simulink model "QuadcopterEMSubs"  (R2023b)
settings: Solver=VariableStepAuto  StartTime=0.0  StopTime=10.0  RelTol=1e-3
libraries: fl_lib x15, nesl_utility x11, sdl_lib x4, ee_lib x4, batteryecm_lib x1
(part 2 of 2)

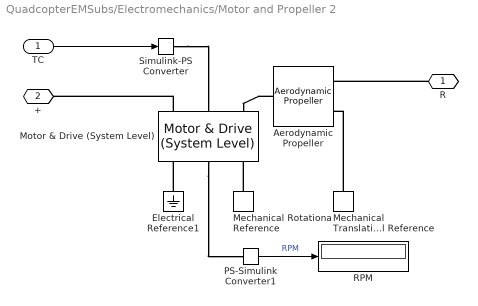
== system QuadcopterEMSubs/Electromechanics/Motor and Propeller 2 ==
  TC : Inport
  Aerodynamic Propeller : sdl_lib/Engines & Motors/Aerodynamic Propeller  parameterization=sdl.enum.PropellerParameterization.Constant  pitch_type=foundation.enum.constant_controlled.constant  direction=sdl.enum.PropellerDirection.Negative  root_pitch=0 deg  D=D m  kt_const=kT  kp_const=kP  kt_poly_fixed=[.002, .0006, -.0509, .0617]  kp_poly_fixed=[-.0752, .0577, -.0622, .16]  pitch_angle_TLU=[-15, 15, 25, 35, 45] deg  kt_poly_TLU=[.0002, -.00041, -.036, .03; .00026, -.00056, -.048, .04; .002, .00063, -.051, .062; .0014, -.0016, -.048, .087; .00087, -.0036, -.041, .12]  kp_poly_TLU=[-.1, .031, .0055, .088; -.081, -.025, .0044, .07; -.075, .058, -.062, .16; -.052, .065, -.08, .3; -.031, .057, -.069, .4]  J_TLU=[.01, .3, .625, 1.55, 2, 2.6]  kt_TLU_1D=[.0614, .0473, .0318, -.0127, -.0343, -.063]  kp_TLU_1D=[.1496, .1314, .116, -.0521, -.1503, -.2813]  kt_TLU_2D=[.00019, .013, .0048, -.017, -.03, -.045; .00039, .025, .0096, -.037, -.06, -.09; .00061, .047, .032, -.013, -.034, -.063; .00086, .072, .057, .014, -.0076, -.036; .12, .104, .09, .049, .029, .0019]  kp_TLU_2D=[.029, .029, .016, .06, .009, -.16; .059, .054, .031, -.12, -.19, -.29; .15, .13, .12, -.052, -.15, -.28; .26, .24, .22, .097, -.04, -.25; .39, .39, .38, .32, .24, .062]  beta_TLU=linspace(0, 360, 10) deg  Ct_TLU_1D=0.035 * sind(linspace(0, 360, 10) - 200)  Cq_TLU_1D=0.010 * sind(linspace(0, 360, 10) - 200)  Ct_TLU_2D=[0.01 * sind(linspace(0, 360, 10) - 200); 0.020 * sind(linspace(0, 360, 10) - 200); 0.035 * sind(linspace(0, 360, 10) - 200); 0.04 * sind(linspace(0, 360, 10) - 200); 0.06 * sind(linspace(0, 360, 10) - 200)]  Cq_TLU_2D=[0.0005 * sind(linspace(0, 360, 10) - 200); 0.0015 * sind(linspace(0, 360, 10) - 200); 0.0025 * sind(linspace(0, 360, 10) - 200); 0.0035 * sind(linspace(0, 360, 10) - 200); 0.0045 * sind(linspace(0, 360, 10) - 200)]  n_blades=2  n_blade_discretization=20  radial_TLU=[.05, .09, .13, .19, .25, .32, .39, .45, .52, .58, .65, .72, 1]  twist_TLU=[48.55, 48.55, 48.55, 48.55, 38.9, 32.39, 27.05, 21.76, 16.74, 12.41, 8.57, 5.52, .034] deg  chord_TLU=[.029, .031, .034, .037, .038, .036, .034, .033, .03, .028, .026, .024, .012]  alpha_TLU=[-180, -169, -161, -143, -39, -28 : -23, -16 : -13, -3, 7 : 17, 21, 35, 36, 60, 120, 144, 160, 169, 180] deg  Cl_TLU=[0, 0, 0, .0038, .0038, .0038, .0044, .0059, .0059, .0063, .0063, .006, .006; 0, 0, 0, .4279, .4367, .4367, .5701, .7465, .7465, .794, .794, .7565, .7565; 0, 0, 0, .6251, .6405, .6405, .6716, .6871, .6871, .6646, .6646, .653, .653; 0, 0, 0, .77, .7939, .7939, .8365, .8507, .8507, .8182, .8182, .8031, .8031; 0, 0, 0, -.8855, -.8888, -.8888, -.8956, -.8987, -.8987, -.8756, -.8756, -.8664, -.8664; 0, 0, 0, -.8164, -.8237, -.8237, -.8446, -.8396, -.8396, -.8173, -.8173, -.8311, -.8311; 0, 0, 0, -.8035, -.8107, -.8107, -.8387, -.8268, -.8268, -.8062, -.8062, -.837, -.837; 0, 0, 0, -.7899, -.7969, -.7969, -.8342, -.8141, -.8141, -.7967, -.7967, -.8448, -.8448; 0, 0, 0, -.7759, -.7829, -.7829, -.8321, -.8021, -.8021, -.7907, -.7907, -.8538, -.8538; 0, 0, 0, -.7597, -.7667, -.7667, -.854, -.7916, -.7916, -.7946, -.7946, -.8715, -.8715; 0, 0, 0, -.7426, -.7496, -.7496, -.8847, -.7891, -.7891, -.8061, -.8061, -.8916, -.8916; 0, 0, 0, -.5682, -.5992, -.5992, -1.2502, -.9071, -.9071, -1.0018, -1.0018, -1.1131, -1.1131; 0, 0, 0, -.5309, -.5773, -.5773, -1.2818, -.9342, -.9342, -1.036, -1.036, -1.1036, -1.1036; 0, 0, 0, -.4907, -.5574, -.5574, -1.2049, -.9612, -.9612, -1.0439, -1.0439, -1.075, -1.075; 0, 0, 0, -.4485, -.5374, -.5374, -1.1187, -.9852, -.9852, -1.0006, -1.0006, -1.0074, -1.0074; 0, 0, 0, .0053, -.2277, -.2277, -.1089, .0596, .0596, .1552, .1552, .0974, .0974; 0, 0, 0, 1.093, 1.1442, 1.1442, 1.2067, 1.2616, 1.2616, 1.2898, 1.2898, 1.1872, 1.1872; 0, 0, 0, 1.2011, 1.2696, 1.2696, 1.3122, 1.3414, 1.3414, 1.3628, 1.3628, 1.2629, 1.2629; 0, 0, 0, 1.2944, 1.3764, 1.3764, 1.3958, 1.4048, 1.4048, 1.4045, 1.4045, 1.331, 1.331; 0, 0, 0, 1.3733, 1.483, 1.483, 1.4631, 1.4421, 1.4421, 1.3507, 1.3507, 1.3853, 1.3853; 0, 0, 0, 1.4289, 1.5767, 1.5767, 1.5156, 1.3648, 1.3648, 1.2843, 1.2843, 1.4168, 1.4168; 0, 0, 0, 1.4765, 1.6474, 1.6474, 1.5515, 1.2718, 1.2718, 1.2722, 1.2722, 1.4354, 1.4354; 0, 0, 0, 1.5166, 1.7035, 1.7035, 1.4574, 1.246, 1.246, 1.273, 1.273, 1.4517, 1.4517; 0, 0, 0, 1.5662, 1.7108, 1.7108, 1.3502, 1.2569, 1.2569, 1.272, 1.272, 1.4472, 1.4472; 0, 0, 0, 1.6172, 1.6861, 1.6861, 1.3319, 1.2727, 1.2727, 1.2756, 1.2756, 1.4453, 1.4453; 0, 0, 0, 1.6518, 1.6448, 1.6448, 1.3288, 1.2899, 1.2899, 1.2853, 1.2853, 1.4478, 1.4478; 0, 0, 0, 1.6837, 1.5939, 1.5939, 1.3215, 1.305, 1.305, 1.3065, 1.3065, 1.4376, 1.4376; 0, 0, 0, 1.8117, 1.5649, 1.5649, 1.4361, 1.359, 1.359, 1.3219, 1.3219, 1.3984, 1.3984; 0, 0, 0, 1.9292, 1.5442, 1.5442, 1.2641, 1.0661, 1.0661, .9471, .9471, .8, .8; 0, 0, 0, 1.9291, 1.5451, 1.5451, 1.2647, 1.0667, 1.0667, .9484, .9484, .8003, .8003; 0, 0, 0, 1.3197, 1.0944, 1.0944, .93, .8084, .8084, .7386, .7386, .6549, .6549; 0, 0, 0, -.5504, -.5764, -.5764, -.5794, -.5974, -.5974, -.6384, -.6384, -.6414, -.6414; 0, 0, 0, -.7967, -.8179, -.8179, -.815, -.8265, -.8265, -.8695, -.8695, -.8727, -.8727; 0, 0, 0, -.6625, -.6755, -.6755, -.6718, -.678, -.678, -.71, -.71, -.7129, -.7129; 0, 0, 0, -.4372, -.4449, -.4449, -.5659, -.7443, -.7443, -.797, -.797, -.7602, -.7602; 0, 0, 0, -.0005, -.0005, -.0005, -.0005, -.0007, -.0007, -.0008, -.0008, -.0007, -.0007]  Cd_TLU=[.5, .5, .35, .0113, .0094, .0094, .0087, .0065, .0065, .0057, .0057, .0052, .0052; .5, .5, .35, .1226, .1192, .1192, .111, .1087, .1087, .1087, .1087, .1096, .1096; .5, .5, .35, .2813, .2754, .2754, .265, .2622, .2622, .2588, .2588, .2588, .2588; .5, .5, .35, .6981, .6956, .6956, .6919, .6916, .6916, .6764, .6764, .6716, .6716; .5, .5, .35, .6005, .6252, .6252, .6685, .6821, .6821, .654, .654, .6398, .6398; .5, .5, .35, .351, .3709, .3709, .4054, .4161, .4161, .3965, .3965, .3833, .3833; .5, .5, .35, .3293, .3486, .3486, .3824, .3927, .3927, .3737, .3737, .3588, .3588; .5, .5, .35, .3079, .3266, .3266, .3597, .3693, .3693, .3508, .3508, .3341, .3341; .5, .5, .35, .2866, .3047, .3047, .3375, .346, .346, .3275, .3275, .3091, .3091; .5, .5, .35, .2658, .2834, .2834, .3163, .3228, .3228, .3033, .3033, .2835, .2835; .5, .5, .35, .2456, .2625, .2625, .2962, .2991, .2991, .2782, .2782, .2577, .2577; .5, .5, .35, .129, .1313, .1313, .1766, .1275, .1275, .096, .096, .0806, .0806; .5, .5, .35, .119, .1157, .1157, .1621, .1039, .1039, .0709, .0709, .0555, .0555; .5, .5, .35, .1107, .1011, .1011, .143, .0807, .0807, .0494, .0494, .0303, .0303; .5, .5, .35, .1041, .0877, .0877, .123, .0586, .0586, .034, .034, .0152, .0152; .5, .5, .35, .0307, .0145, .0145, .0089, .0068, .0068, .0058, .0058, .0065, .0065; .5, .5, .35, .0156, .0115, .0115, .0106, .013, .013, .013, .013, .0112, .0112; .5, .5, .35, .0194, .0119, .0119, .0123, .0151, .0151, .0146, .0146, .0123, .0123; .5, .5, .35, .0268, .0132, .0132, .0153, .0178, .0178, .0177, .0177, .0135, .0135; .5, .5, .35, .0381, .0154, .0154, .0188, .0252, .0252, .0248, .0248, .0148, .0148; .5, .5, .35, .0563, .019, .019, .0248, .0406, .0406, .0339, .0339, .0365, .0365; .5, .5, .35, .0794, .0262, .0262, .0359, .0587, .0587, .0457, .0457, .0595, .0595; .5, .5, .35, .1104, .0384, .0384, .0602, .077, .077, .0619, .0619, .0823, .0823; .5, .5, .35, .1435, .0591, .0591, .0907, .0982, .0982, .0792, .0792, .1047, .1047; .5, .5, .35, .1813, .0944, .0944, .1213, .1201, .1201, .0973, .0973, .1269, .1269; .5, .5, .35, .2217, .1343, .1343, .1565, .1416, .1416, .1154, .1154, .1491, .1491; .5, .5, .35, .2649, .1779, .1779, .1878, .1632, .1632, .1352, .1352, .1711, .1711; .5, .5, .35, .4382, .3418, .3418, .2921, .2513, .2513, .2194, .2194, .2573, .2573; .5, .5, .35, 1.0687, .884, .884, .7413, .6526, .6526, .6107, .6107, .5307, .5307; .5, .5, .35, 1.1128, .9207, .9207, .7724, .6799, .6799, .6362, .6362, .5527, .5527; .5, .5, .35, 1.8354, 1.5718, 1.5718, 1.3636, 1.232, 1.232, 1.1782, 1.1782, 1.0678, 1.0678; .5, .5, .35, 1.1876, 1.1903, 1.1903, 1.1775, 1.1722, 1.1722, 1.207, 1.207, 1.2112, 1.2112; .5, .5, .35, .7009, .6946, .6946, .6841, .6742, .6742, .6875, .6875, .6898, .6898; .5, .5, .35, .3164, .3083, .3083, .3017, .2929, .2929, .2939, .2939, .2948, .2948; .5, .5, .35, .1294, .1254, .1254, .1229, .1168, .1168, .1143, .1143, .1146, .1146; .5, .5, .35, .0601, .0405, .0405, .0265, .0201, .0201, .0184, .0184, .0197, .0197]  interp_method=simscape.enum.interpolation.linear  extrap_method=simscape.enum.extrapolation.linear  density_spec=foundation.enum.constant_variable.constant  rho=1.225 kg/m^3  rotational_ports=sdl.enum.ConnectionType.Conserving  translational_ports=sdl.enum.ConnectionType.Conserving  model_inertia=true  propeller_inertia=J kg*m^2  propeller_mass=m g  efficiency_sensor=false  n_thr=0.001 Hz  k_thr=0.001  P_thr=0.01 W  operation_check=simscape.enum.assert.action.warn  expose_port_C=0  w_specify=off  w_priority=None  w=0 rad/s  w_nominal_specify=off  w_nominal_unit=rad/s  w_nominal_value=1  Q_specify=off  Q_priority=None  Q=0 N*m  Q_nominal_specify=off  Q_nominal_unit=N*m  Q_nominal_value=1  v_specify=off  v_priority=None  v=0 m/s  v_nominal_specify=off  v_nominal_unit=m/s  v_nominal_value=1  thrust_specify=off  thrust_priority=None  thrust=0 N  thrust_nominal_specify=off  thrust_nominal_unit=N  thrust_nominal_value=1
      settings: InternalSimscapePortConfiguration="{\"Bottom\":[],\"Left\":[{\"id\":\"R1\",\"label\":\"R1\",\"type\":\"foundation.mechanical.rotational.rotational\"}],\"Right\":[{\"id\":\"R2\",\"label\":\"R2\",\"type\":\"foundation.mechanical.translational.translational\"},{\"id\":\"C2\",\"label\":\"C2\",\"type\":\"foundation.mechanical.translational.translational\"}],\"Top\":[]}"
  Electrical Reference1 : fl_lib/Electrical/Electrical Elements/Electrical Reference
  Mechanical Rotational Reference : fl_lib/Mechanical/Rotational Elements/Mechanical Rotational Reference
  Mechanical Translational Reference : fl_lib/Mechanical/Translational Elements/Mechanical Translational Reference
  Motor & Drive (System Level) : ee_lib/Electromechanical/Motor & Drive (System Level)  torque_speed_param=ee.enum.electromech.envelope.torque_power  overtorque_param=ee.enum.electromech.overtorque.no  T_t=[.09, .08, .07, 0] N*m  T_t_intermittent=[.36, .32, .28, 0] N*m  T_t_2D=[.09, .09, .09; .08, .08, .08; .07, .07, .07; 0, 0, 0] N*m  T_t_intermittent_2D=[.36, .36, .36; .32, .32, .32; .28, .28, .28; 0, 0, 0] N*m  w_t=[0, 3750, 7500, 8000] rpm  vdc_t=[6, 12, 24] V  torque_max=1 mN*m  power_max=3 W  torque_max_intermittent=0.4 N*m  power_max_intermittent=120 W  time_overtorque=30 s  time_recover=60 s  Tc=0.02 s  EnableSwitch=simscape.enum.onoff.off  losses_param=1  eff=74  w_eff=3e4 rpm  T_eff=1 mN*m  Piron=0 W  Pbase=0 W  w_eff_vec=[-8000, -4000, 0, 4000, 8000] rpm  T_eff_vec=[0, .03, .06, .09] N*m  v_eff_vec=[100, 250, 400] V  losses_mat=[1.49, 1.67, 2.21, 3.1; .42, .69, 1.14, 2.03; .06, .24, .78, 1.68; .42, .69, 1.14, 2.03; 1.49, 1.67, 2.21, 3.1] W  efficiency_mat=[95, 95, 95, 95; 95, 95, 95, 95; 95, 95, 95, 95; 95, 95, 95, 95; 95, 95, 95, 95]  losses_mat_3D=ones(5, 4, 3) W  efficiency_mat_3D=95 * ones(5, 4, 3)  Res=0 Ohm  enable_fault=simscape.enum.onoff.off  fault_condition=1  fault_threshold=0.5  J=8e-9 kg*m^2  lam=2.5e-8 N*m*s/rad  speed0=0 rpm  faulted_specify=off  faulted_priority=None  faulted=0  faulted_nominal_specify=off  faulted_nominal_unit=1  faulted_nominal_value=1  isSwitchedOff_specify=off  isSwitchedOff_priority=None  isSwitchedOff=0  isSwitchedOff_nominal_specify=off  isSwitchedOff_nominal_unit=1  isSwitchedOff_nominal_value=1  torqueLimitContinuous_specify=off  torqueLimitContinuous_priority=None  torqueLimitContinuous=0 N*m  torqueLimitContinuous_nominal_specify=off  torqueLimitContinuous_nominal_unit=N*m  torqueLimitContinuous_nominal_value=1  alpha=3.93e-3 1/K  Tmeas=25 degC  Tmeas2=125 degC  losses_mat_T2=[1.49, 1.74, 2.49, 3.74; .42, .67, 1.42, 2.67; .06, .31, 1.06, 2.31; .42, .67, 1.42, 2.67; 1.49, 1.74, 2.49, 3.74] W  efficiency_mat_T2=[95, 95, 95, 95; 95, 95, 95, 95; 95, 95, 95, 95; 95, 95, 95, 95; 95, 95, 95, 95]  losses_mat_3D_T2=ones(5, 4, 3) W  efficiency_mat_3D_T2=95 * ones(5, 4, 3)  thermal_mass=100 J/K  initial_temperature=25 degC
  PS-Simulink Converter1 : nesl_utility/PS-Simulink Converter  PhysicalDomain=network_engine_domain  SubClassName=ps_output  LeftPortType=input  RightPortType=output  PseudoPeriodic=off  Frequencies=[]  VectorFormat=inherit  Unit=rpm  AffineConversion=off
  RPM : Display
  Simulink-PS Converter : nesl_utility/Simulink-PS Converter  PhysicalDomain=network_engine_domain  SubClassName=ps_input  LeftPortType=input  RightPortType=output  PseudoPeriodic=off  Frequencies=[]  NoiseDistribution=none  NoiseParameters=[]  Unit=mN*m  AffineConversion=off  FilteringAndDerivatives=provide  SimscapeFilterOrder=1  InputFilterTimeConstant=0.001  UdotUserProvided=0
  R : PMIOPort  Side=Right
  + : PMIOPort  Port=2  Side=Left
  wires:
  TC/1 -> Simulink-PS Converter/1
  PS-Simulink Converter1/1 -> RPM/1  "RPM"
  connections:
  Mechanical Rotational Reference/LConn1 -- Motor & Drive (System Level)/RConn3
  Electrical Reference1/LConn1 -- Motor & Drive (System Level)/RConn1
  Aerodynamic Propeller/LConn1 -- Motor & Drive (System Level)/LConn3
  Motor & Drive (System Level)/RConn2 -- PS-Simulink Converter1/LConn1
  Mechanical Translational Reference/LConn1 -- Aerodynamic Propeller/RConn2
  R/RConn1 -- Aerodynamic Propeller/RConn1
  Simulink-PS Converter/RConn1 -- Motor & Drive (System Level)/LConn2
  Motor & Drive (System Level)/LConn1 -- +/RConn1

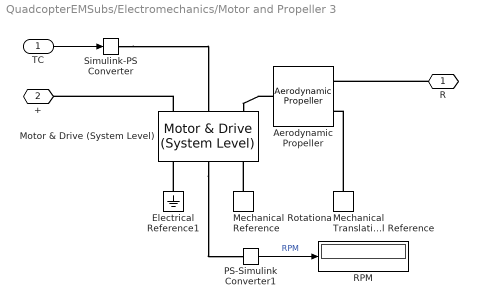
== system QuadcopterEMSubs/Electromechanics/Motor and Propeller 3 ==
  TC : Inport
  Aerodynamic Propeller : sdl_lib/Engines & Motors/Aerodynamic Propeller  parameterization=sdl.enum.PropellerParameterization.Constant  pitch_type=foundation.enum.constant_controlled.constant  direction=sdl.enum.PropellerDirection.Positive  root_pitch=0 deg  D=D m  kt_const=kT  kp_const=kP  kt_poly_fixed=[.002, .0006, -.0509, .0617]  kp_poly_fixed=[-.0752, .0577, -.0622, .16]  pitch_angle_TLU=[-15, 15, 25, 35, 45] deg  kt_poly_TLU=[.0002, -.00041, -.036, .03; .00026, -.00056, -.048, .04; .002, .00063, -.051, .062; .0014, -.0016, -.048, .087; .00087, -.0036, -.041, .12]  kp_poly_TLU=[-.1, .031, .0055, .088; -.081, -.025, .0044, .07; -.075, .058, -.062, .16; -.052, .065, -.08, .3; -.031, .057, -.069, .4]  J_TLU=[.01, .3, .625, 1.55, 2, 2.6]  kt_TLU_1D=[.0614, .0473, .0318, -.0127, -.0343, -.063]  kp_TLU_1D=[.1496, .1314, .116, -.0521, -.1503, -.2813]  kt_TLU_2D=[.00019, .013, .0048, -.017, -.03, -.045; .00039, .025, .0096, -.037, -.06, -.09; .00061, .047, .032, -.013, -.034, -.063; .00086, .072, .057, .014, -.0076, -.036; .12, .104, .09, .049, .029, .0019]  kp_TLU_2D=[.029, .029, .016, .06, .009, -.16; .059, .054, .031, -.12, -.19, -.29; .15, .13, .12, -.052, -.15, -.28; .26, .24, .22, .097, -.04, -.25; .39, .39, .38, .32, .24, .062]  beta_TLU=linspace(0, 360, 10) deg  Ct_TLU_1D=0.035 * sind(linspace(0, 360, 10) - 200)  Cq_TLU_1D=0.010 * sind(linspace(0, 360, 10) - 200)  Ct_TLU_2D=[0.01 * sind(linspace(0, 360, 10) - 200); 0.020 * sind(linspace(0, 360, 10) - 200); 0.035 * sind(linspace(0, 360, 10) - 200); 0.04 * sind(linspace(0, 360, 10) - 200); 0.06 * sind(linspace(0, 360, 10) - 200)]  Cq_TLU_2D=[0.0005 * sind(linspace(0, 360, 10) - 200); 0.0015 * sind(linspace(0, 360, 10) - 200); 0.0025 * sind(linspace(0, 360, 10) - 200); 0.0035 * sind(linspace(0, 360, 10) - 200); 0.0045 * sind(linspace(0, 360, 10) - 200)]  n_blades=2  n_blade_discretization=20  radial_TLU=[.05, .09, .13, .19, .25, .32, .39, .45, .52, .58, .65, .72, 1]  twist_TLU=[48.55, 48.55, 48.55, 48.55, 38.9, 32.39, 27.05, 21.76, 16.74, 12.41, 8.57, 5.52, .034] deg  chord_TLU=[.029, .031, .034, .037, .038, .036, .034, .033, .03, .028, .026, .024, .012]  alpha_TLU=[-180, -169, -161, -143, -39, -28 : -23, -16 : -13, -3, 7 : 17, 21, 35, 36, 60, 120, 144, 160, 169, 180] deg  Cl_TLU=[0, 0, 0, .0038, .0038, .0038, .0044, .0059, .0059, .0063, .0063, .006, .006; 0, 0, 0, .4279, .4367, .4367, .5701, .7465, .7465, .794, .794, .7565, .7565; 0, 0, 0, .6251, .6405, .6405, .6716, .6871, .6871, .6646, .6646, .653, .653; 0, 0, 0, .77, .7939, .7939, .8365, .8507, .8507, .8182, .8182, .8031, .8031; 0, 0, 0, -.8855, -.8888, -.8888, -.8956, -.8987, -.8987, -.8756, -.8756, -.8664, -.8664; 0, 0, 0, -.8164, -.8237, -.8237, -.8446, -.8396, -.8396, -.8173, -.8173, -.8311, -.8311; 0, 0, 0, -.8035, -.8107, -.8107, -.8387, -.8268, -.8268, -.8062, -.8062, -.837, -.837; 0, 0, 0, -.7899, -.7969, -.7969, -.8342, -.8141, -.8141, -.7967, -.7967, -.8448, -.8448; 0, 0, 0, -.7759, -.7829, -.7829, -.8321, -.8021, -.8021, -.7907, -.7907, -.8538, -.8538; 0, 0, 0, -.7597, -.7667, -.7667, -.854, -.7916, -.7916, -.7946, -.7946, -.8715, -.8715; 0, 0, 0, -.7426, -.7496, -.7496, -.8847, -.7891, -.7891, -.8061, -.8061, -.8916, -.8916; 0, 0, 0, -.5682, -.5992, -.5992, -1.2502, -.9071, -.9071, -1.0018, -1.0018, -1.1131, -1.1131; 0, 0, 0, -.5309, -.5773, -.5773, -1.2818, -.9342, -.9342, -1.036, -1.036, -1.1036, -1.1036; 0, 0, 0, -.4907, -.5574, -.5574, -1.2049, -.9612, -.9612, -1.0439, -1.0439, -1.075, -1.075; 0, 0, 0, -.4485, -.5374, -.5374, -1.1187, -.9852, -.9852, -1.0006, -1.0006, -1.0074, -1.0074; 0, 0, 0, .0053, -.2277, -.2277, -.1089, .0596, .0596, .1552, .1552, .0974, .0974; 0, 0, 0, 1.093, 1.1442, 1.1442, 1.2067, 1.2616, 1.2616, 1.2898, 1.2898, 1.1872, 1.1872; 0, 0, 0, 1.2011, 1.2696, 1.2696, 1.3122, 1.3414, 1.3414, 1.3628, 1.3628, 1.2629, 1.2629; 0, 0, 0, 1.2944, 1.3764, 1.3764, 1.3958, 1.4048, 1.4048, 1.4045, 1.4045, 1.331, 1.331; 0, 0, 0, 1.3733, 1.483, 1.483, 1.4631, 1.4421, 1.4421, 1.3507, 1.3507, 1.3853, 1.3853; 0, 0, 0, 1.4289, 1.5767, 1.5767, 1.5156, 1.3648, 1.3648, 1.2843, 1.2843, 1.4168, 1.4168; 0, 0, 0, 1.4765, 1.6474, 1.6474, 1.5515, 1.2718, 1.2718, 1.2722, 1.2722, 1.4354, 1.4354; 0, 0, 0, 1.5166, 1.7035, 1.7035, 1.4574, 1.246, 1.246, 1.273, 1.273, 1.4517, 1.4517; 0, 0, 0, 1.5662, 1.7108, 1.7108, 1.3502, 1.2569, 1.2569, 1.272, 1.272, 1.4472, 1.4472; 0, 0, 0, 1.6172, 1.6861, 1.6861, 1.3319, 1.2727, 1.2727, 1.2756, 1.2756, 1.4453, 1.4453; 0, 0, 0, 1.6518, 1.6448, 1.6448, 1.3288, 1.2899, 1.2899, 1.2853, 1.2853, 1.4478, 1.4478; 0, 0, 0, 1.6837, 1.5939, 1.5939, 1.3215, 1.305, 1.305, 1.3065, 1.3065, 1.4376, 1.4376; 0, 0, 0, 1.8117, 1.5649, 1.5649, 1.4361, 1.359, 1.359, 1.3219, 1.3219, 1.3984, 1.3984; 0, 0, 0, 1.9292, 1.5442, 1.5442, 1.2641, 1.0661, 1.0661, .9471, .9471, .8, .8; 0, 0, 0, 1.9291, 1.5451, 1.5451, 1.2647, 1.0667, 1.0667, .9484, .9484, .8003, .8003; 0, 0, 0, 1.3197, 1.0944, 1.0944, .93, .8084, .8084, .7386, .7386, .6549, .6549; 0, 0, 0, -.5504, -.5764, -.5764, -.5794, -.5974, -.5974, -.6384, -.6384, -.6414, -.6414; 0, 0, 0, -.7967, -.8179, -.8179, -.815, -.8265, -.8265, -.8695, -.8695, -.8727, -.8727; 0, 0, 0, -.6625, -.6755, -.6755, -.6718, -.678, -.678, -.71, -.71, -.7129, -.7129; 0, 0, 0, -.4372, -.4449, -.4449, -.5659, -.7443, -.7443, -.797, -.797, -.7602, -.7602; 0, 0, 0, -.0005, -.0005, -.0005, -.0005, -.0007, -.0007, -.0008, -.0008, -.0007, -.0007]  Cd_TLU=[.5, .5, .35, .0113, .0094, .0094, .0087, .0065, .0065, .0057, .0057, .0052, .0052; .5, .5, .35, .1226, .1192, .1192, .111, .1087, .1087, .1087, .1087, .1096, .1096; .5, .5, .35, .2813, .2754, .2754, .265, .2622, .2622, .2588, .2588, .2588, .2588; .5, .5, .35, .6981, .6956, .6956, .6919, .6916, .6916, .6764, .6764, .6716, .6716; .5, .5, .35, .6005, .6252, .6252, .6685, .6821, .6821, .654, .654, .6398, .6398; .5, .5, .35, .351, .3709, .3709, .4054, .4161, .4161, .3965, .3965, .3833, .3833; .5, .5, .35, .3293, .3486, .3486, .3824, .3927, .3927, .3737, .3737, .3588, .3588; .5, .5, .35, .3079, .3266, .3266, .3597, .3693, .3693, .3508, .3508, .3341, .3341; .5, .5, .35, .2866, .3047, .3047, .3375, .346, .346, .3275, .3275, .3091, .3091; .5, .5, .35, .2658, .2834, .2834, .3163, .3228, .3228, .3033, .3033, .2835, .2835; .5, .5, .35, .2456, .2625, .2625, .2962, .2991, .2991, .2782, .2782, .2577, .2577; .5, .5, .35, .129, .1313, .1313, .1766, .1275, .1275, .096, .096, .0806, .0806; .5, .5, .35, .119, .1157, .1157, .1621, .1039, .1039, .0709, .0709, .0555, .0555; .5, .5, .35, .1107, .1011, .1011, .143, .0807, .0807, .0494, .0494, .0303, .0303; .5, .5, .35, .1041, .0877, .0877, .123, .0586, .0586, .034, .034, .0152, .0152; .5, .5, .35, .0307, .0145, .0145, .0089, .0068, .0068, .0058, .0058, .0065, .0065; .5, .5, .35, .0156, .0115, .0115, .0106, .013, .013, .013, .013, .0112, .0112; .5, .5, .35, .0194, .0119, .0119, .0123, .0151, .0151, .0146, .0146, .0123, .0123; .5, .5, .35, .0268, .0132, .0132, .0153, .0178, .0178, .0177, .0177, .0135, .0135; .5, .5, .35, .0381, .0154, .0154, .0188, .0252, .0252, .0248, .0248, .0148, .0148; .5, .5, .35, .0563, .019, .019, .0248, .0406, .0406, .0339, .0339, .0365, .0365; .5, .5, .35, .0794, .0262, .0262, .0359, .0587, .0587, .0457, .0457, .0595, .0595; .5, .5, .35, .1104, .0384, .0384, .0602, .077, .077, .0619, .0619, .0823, .0823; .5, .5, .35, .1435, .0591, .0591, .0907, .0982, .0982, .0792, .0792, .1047, .1047; .5, .5, .35, .1813, .0944, .0944, .1213, .1201, .1201, .0973, .0973, .1269, .1269; .5, .5, .35, .2217, .1343, .1343, .1565, .1416, .1416, .1154, .1154, .1491, .1491; .5, .5, .35, .2649, .1779, .1779, .1878, .1632, .1632, .1352, .1352, .1711, .1711; .5, .5, .35, .4382, .3418, .3418, .2921, .2513, .2513, .2194, .2194, .2573, .2573; .5, .5, .35, 1.0687, .884, .884, .7413, .6526, .6526, .6107, .6107, .5307, .5307; .5, .5, .35, 1.1128, .9207, .9207, .7724, .6799, .6799, .6362, .6362, .5527, .5527; .5, .5, .35, 1.8354, 1.5718, 1.5718, 1.3636, 1.232, 1.232, 1.1782, 1.1782, 1.0678, 1.0678; .5, .5, .35, 1.1876, 1.1903, 1.1903, 1.1775, 1.1722, 1.1722, 1.207, 1.207, 1.2112, 1.2112; .5, .5, .35, .7009, .6946, .6946, .6841, .6742, .6742, .6875, .6875, .6898, .6898; .5, .5, .35, .3164, .3083, .3083, .3017, .2929, .2929, .2939, .2939, .2948, .2948; .5, .5, .35, .1294, .1254, .1254, .1229, .1168, .1168, .1143, .1143, .1146, .1146; .5, .5, .35, .0601, .0405, .0405, .0265, .0201, .0201, .0184, .0184, .0197, .0197]  interp_method=simscape.enum.interpolation.linear  extrap_method=simscape.enum.extrapolation.linear  density_spec=foundation.enum.constant_variable.constant  rho=1.225 kg/m^3  rotational_ports=sdl.enum.ConnectionType.Conserving  translational_ports=sdl.enum.ConnectionType.Conserving  model_inertia=true  propeller_inertia=J kg*m^2  propeller_mass=m g  efficiency_sensor=false  n_thr=0.001 Hz  k_thr=0.001  P_thr=0.01 W  operation_check=simscape.enum.assert.action.warn  expose_port_C=0  w_specify=off  w_priority=None  w=0 rad/s  w_nominal_specify=off  w_nominal_unit=rad/s  w_nominal_value=1  Q_specify=off  Q_priority=None  Q=0 N*m  Q_nominal_specify=off  Q_nominal_unit=N*m  Q_nominal_value=1  v_specify=off  v_priority=None  v=0 m/s  v_nominal_specify=off  v_nominal_unit=m/s  v_nominal_value=1  thrust_specify=off  thrust_priority=None  thrust=0 N  thrust_nominal_specify=off  thrust_nominal_unit=N  thrust_nominal_value=1
      settings: InternalSimscapePortConfiguration="{\"Bottom\":[],\"Left\":[{\"id\":\"R1\",\"label\":\"R1\",\"type\":\"foundation.mechanical.rotational.rotational\"}],\"Right\":[{\"id\":\"R2\",\"label\":\"R2\",\"type\":\"foundation.mechanical.translational.translational\"},{\"id\":\"C2\",\"label\":\"C2\",\"type\":\"foundation.mechanical.translational.translational\"}],\"Top\":[]}"
  Electrical Reference1 : fl_lib/Electrical/Electrical Elements/Electrical Reference
  Mechanical Rotational Reference : fl_lib/Mechanical/Rotational Elements/Mechanical Rotational Reference
  Mechanical Translational Reference : fl_lib/Mechanical/Translational Elements/Mechanical Translational Reference
  Motor & Drive (System Level) : ee_lib/Electromechanical/Motor & Drive (System Level)  torque_speed_param=ee.enum.electromech.envelope.torque_power  overtorque_param=ee.enum.electromech.overtorque.no  T_t=[.09, .08, .07, 0] N*m  T_t_intermittent=[.36, .32, .28, 0] N*m  T_t_2D=[.09, .09, .09; .08, .08, .08; .07, .07, .07; 0, 0, 0] N*m  T_t_intermittent_2D=[.36, .36, .36; .32, .32, .32; .28, .28, .28; 0, 0, 0] N*m  w_t=[0, 3750, 7500, 8000] rpm  vdc_t=[6, 12, 24] V  torque_max=1 mN*m  power_max=3 W  torque_max_intermittent=0.4 N*m  power_max_intermittent=120 W  time_overtorque=30 s  time_recover=60 s  Tc=0.02 s  EnableSwitch=simscape.enum.onoff.off  losses_param=1  eff=74  w_eff=3e4 rpm  T_eff=1 mN*m  Piron=0 W  Pbase=0 W  w_eff_vec=[-8000, -4000, 0, 4000, 8000] rpm  T_eff_vec=[0, .03, .06, .09] N*m  v_eff_vec=[100, 250, 400] V  losses_mat=[1.49, 1.67, 2.21, 3.1; .42, .69, 1.14, 2.03; .06, .24, .78, 1.68; .42, .69, 1.14, 2.03; 1.49, 1.67, 2.21, 3.1] W  efficiency_mat=[95, 95, 95, 95; 95, 95, 95, 95; 95, 95, 95, 95; 95, 95, 95, 95; 95, 95, 95, 95]  losses_mat_3D=ones(5, 4, 3) W  efficiency_mat_3D=95 * ones(5, 4, 3)  Res=0 Ohm  enable_fault=simscape.enum.onoff.off  fault_condition=1  fault_threshold=0.5  J=8e-9 kg*m^2  lam=2.5e-8 N*m*s/rad  speed0=0 rpm  faulted_specify=off  faulted_priority=None  faulted=0  faulted_nominal_specify=off  faulted_nominal_unit=1  faulted_nominal_value=1  isSwitchedOff_specify=off  isSwitchedOff_priority=None  isSwitchedOff=0  isSwitchedOff_nominal_specify=off  isSwitchedOff_nominal_unit=1  isSwitchedOff_nominal_value=1  torqueLimitContinuous_specify=off  torqueLimitContinuous_priority=None  torqueLimitContinuous=0 N*m  torqueLimitContinuous_nominal_specify=off  torqueLimitContinuous_nominal_unit=N*m  torqueLimitContinuous_nominal_value=1  alpha=3.93e-3 1/K  Tmeas=25 degC  Tmeas2=125 degC  losses_mat_T2=[1.49, 1.74, 2.49, 3.74; .42, .67, 1.42, 2.67; .06, .31, 1.06, 2.31; .42, .67, 1.42, 2.67; 1.49, 1.74, 2.49, 3.74] W  efficiency_mat_T2=[95, 95, 95, 95; 95, 95, 95, 95; 95, 95, 95, 95; 95, 95, 95, 95; 95, 95, 95, 95]  losses_mat_3D_T2=ones(5, 4, 3) W  efficiency_mat_3D_T2=95 * ones(5, 4, 3)  thermal_mass=100 J/K  initial_temperature=25 degC
  PS-Simulink Converter1 : nesl_utility/PS-Simulink Converter  PhysicalDomain=network_engine_domain  SubClassName=ps_output  LeftPortType=input  RightPortType=output  PseudoPeriodic=off  Frequencies=[]  VectorFormat=inherit  Unit=rpm  AffineConversion=off
  RPM : Display
  Simulink-PS Converter : nesl_utility/Simulink-PS Converter  PhysicalDomain=network_engine_domain  SubClassName=ps_input  LeftPortType=input  RightPortType=output  PseudoPeriodic=off  Frequencies=[]  NoiseDistribution=none  NoiseParameters=[]  Unit=mN*m  AffineConversion=off  FilteringAndDerivatives=provide  SimscapeFilterOrder=1  InputFilterTimeConstant=0.001  UdotUserProvided=0
  R : PMIOPort  Side=Right
  + : PMIOPort  Port=2  Side=Left
  wires:
  PS-Simulink Converter1/1 -> RPM/1  "RPM"
  TC/1 -> Simulink-PS Converter/1
  connections:
  Mechanical Rotational Reference/LConn1 -- Motor & Drive (System Level)/RConn3
  Electrical Reference1/LConn1 -- Motor & Drive (System Level)/RConn1
  Aerodynamic Propeller/LConn1 -- Motor & Drive (System Level)/LConn3
  Motor & Drive (System Level)/RConn2 -- PS-Simulink Converter1/LConn1
  Mechanical Translational Reference/LConn1 -- Aerodynamic Propeller/RConn2
  R/RConn1 -- Aerodynamic Propeller/RConn1
  Simulink-PS Converter/RConn1 -- Motor & Drive (System Level)/LConn2
  Motor & Drive (System Level)/LConn1 -- +/RConn1

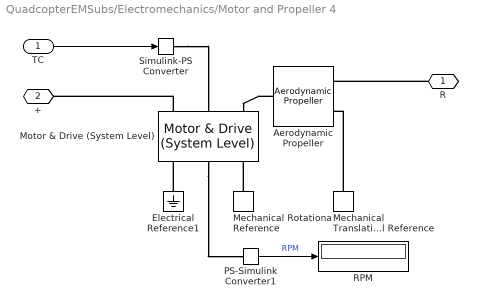
== system QuadcopterEMSubs/Electromechanics/Motor and Propeller 4 ==
  TC : Inport
  Aerodynamic Propeller : sdl_lib/Engines & Motors/Aerodynamic Propeller  parameterization=sdl.enum.PropellerParameterization.Constant  pitch_type=foundation.enum.constant_controlled.constant  direction=sdl.enum.PropellerDirection.Negative  root_pitch=0 deg  D=D m  kt_const=kT  kp_const=kP  kt_poly_fixed=[.002, .0006, -.0509, .0617]  kp_poly_fixed=[-.0752, .0577, -.0622, .16]  pitch_angle_TLU=[-15, 15, 25, 35, 45] deg  kt_poly_TLU=[.0002, -.00041, -.036, .03; .00026, -.00056, -.048, .04; .002, .00063, -.051, .062; .0014, -.0016, -.048, .087; .00087, -.0036, -.041, .12]  kp_poly_TLU=[-.1, .031, .0055, .088; -.081, -.025, .0044, .07; -.075, .058, -.062, .16; -.052, .065, -.08, .3; -.031, .057, -.069, .4]  J_TLU=[.01, .3, .625, 1.55, 2, 2.6]  kt_TLU_1D=[.0614, .0473, .0318, -.0127, -.0343, -.063]  kp_TLU_1D=[.1496, .1314, .116, -.0521, -.1503, -.2813]  kt_TLU_2D=[.00019, .013, .0048, -.017, -.03, -.045; .00039, .025, .0096, -.037, -.06, -.09; .00061, .047, .032, -.013, -.034, -.063; .00086, .072, .057, .014, -.0076, -.036; .12, .104, .09, .049, .029, .0019]  kp_TLU_2D=[.029, .029, .016, .06, .009, -.16; .059, .054, .031, -.12, -.19, -.29; .15, .13, .12, -.052, -.15, -.28; .26, .24, .22, .097, -.04, -.25; .39, .39, .38, .32, .24, .062]  beta_TLU=linspace(0, 360, 10) deg  Ct_TLU_1D=0.035 * sind(linspace(0, 360, 10) - 200)  Cq_TLU_1D=0.010 * sind(linspace(0, 360, 10) - 200)  Ct_TLU_2D=[0.01 * sind(linspace(0, 360, 10) - 200); 0.020 * sind(linspace(0, 360, 10) - 200); 0.035 * sind(linspace(0, 360, 10) - 200); 0.04 * sind(linspace(0, 360, 10) - 200); 0.06 * sind(linspace(0, 360, 10) - 200)]  Cq_TLU_2D=[0.0005 * sind(linspace(0, 360, 10) - 200); 0.0015 * sind(linspace(0, 360, 10) - 200); 0.0025 * sind(linspace(0, 360, 10) - 200); 0.0035 * sind(linspace(0, 360, 10) - 200); 0.0045 * sind(linspace(0, 360, 10) - 200)]  n_blades=2  n_blade_discretization=20  radial_TLU=[.05, .09, .13, .19, .25, .32, .39, .45, .52, .58, .65, .72, 1]  twist_TLU=[48.55, 48.55, 48.55, 48.55, 38.9, 32.39, 27.05, 21.76, 16.74, 12.41, 8.57, 5.52, .034] deg  chord_TLU=[.029, .031, .034, .037, .038, .036, .034, .033, .03, .028, .026, .024, .012]  alpha_TLU=[-180, -169, -161, -143, -39, -28 : -23, -16 : -13, -3, 7 : 17, 21, 35, 36, 60, 120, 144, 160, 169, 180] deg  Cl_TLU=[0, 0, 0, .0038, .0038, .0038, .0044, .0059, .0059, .0063, .0063, .006, .006; 0, 0, 0, .4279, .4367, .4367, .5701, .7465, .7465, .794, .794, .7565, .7565; 0, 0, 0, .6251, .6405, .6405, .6716, .6871, .6871, .6646, .6646, .653, .653; 0, 0, 0, .77, .7939, .7939, .8365, .8507, .8507, .8182, .8182, .8031, .8031; 0, 0, 0, -.8855, -.8888, -.8888, -.8956, -.8987, -.8987, -.8756, -.8756, -.8664, -.8664; 0, 0, 0, -.8164, -.8237, -.8237, -.8446, -.8396, -.8396, -.8173, -.8173, -.8311, -.8311; 0, 0, 0, -.8035, -.8107, -.8107, -.8387, -.8268, -.8268, -.8062, -.8062, -.837, -.837; 0, 0, 0, -.7899, -.7969, -.7969, -.8342, -.8141, -.8141, -.7967, -.7967, -.8448, -.8448; 0, 0, 0, -.7759, -.7829, -.7829, -.8321, -.8021, -.8021, -.7907, -.7907, -.8538, -.8538; 0, 0, 0, -.7597, -.7667, -.7667, -.854, -.7916, -.7916, -.7946, -.7946, -.8715, -.8715; 0, 0, 0, -.7426, -.7496, -.7496, -.8847, -.7891, -.7891, -.8061, -.8061, -.8916, -.8916; 0, 0, 0, -.5682, -.5992, -.5992, -1.2502, -.9071, -.9071, -1.0018, -1.0018, -1.1131, -1.1131; 0, 0, 0, -.5309, -.5773, -.5773, -1.2818, -.9342, -.9342, -1.036, -1.036, -1.1036, -1.1036; 0, 0, 0, -.4907, -.5574, -.5574, -1.2049, -.9612, -.9612, -1.0439, -1.0439, -1.075, -1.075; 0, 0, 0, -.4485, -.5374, -.5374, -1.1187, -.9852, -.9852, -1.0006, -1.0006, -1.0074, -1.0074; 0, 0, 0, .0053, -.2277, -.2277, -.1089, .0596, .0596, .1552, .1552, .0974, .0974; 0, 0, 0, 1.093, 1.1442, 1.1442, 1.2067, 1.2616, 1.2616, 1.2898, 1.2898, 1.1872, 1.1872; 0, 0, 0, 1.2011, 1.2696, 1.2696, 1.3122, 1.3414, 1.3414, 1.3628, 1.3628, 1.2629, 1.2629; 0, 0, 0, 1.2944, 1.3764, 1.3764, 1.3958, 1.4048, 1.4048, 1.4045, 1.4045, 1.331, 1.331; 0, 0, 0, 1.3733, 1.483, 1.483, 1.4631, 1.4421, 1.4421, 1.3507, 1.3507, 1.3853, 1.3853; 0, 0, 0, 1.4289, 1.5767, 1.5767, 1.5156, 1.3648, 1.3648, 1.2843, 1.2843, 1.4168, 1.4168; 0, 0, 0, 1.4765, 1.6474, 1.6474, 1.5515, 1.2718, 1.2718, 1.2722, 1.2722, 1.4354, 1.4354; 0, 0, 0, 1.5166, 1.7035, 1.7035, 1.4574, 1.246, 1.246, 1.273, 1.273, 1.4517, 1.4517; 0, 0, 0, 1.5662, 1.7108, 1.7108, 1.3502, 1.2569, 1.2569, 1.272, 1.272, 1.4472, 1.4472; 0, 0, 0, 1.6172, 1.6861, 1.6861, 1.3319, 1.2727, 1.2727, 1.2756, 1.2756, 1.4453, 1.4453; 0, 0, 0, 1.6518, 1.6448, 1.6448, 1.3288, 1.2899, 1.2899, 1.2853, 1.2853, 1.4478, 1.4478; 0, 0, 0, 1.6837, 1.5939, 1.5939, 1.3215, 1.305, 1.305, 1.3065, 1.3065, 1.4376, 1.4376; 0, 0, 0, 1.8117, 1.5649, 1.5649, 1.4361, 1.359, 1.359, 1.3219, 1.3219, 1.3984, 1.3984; 0, 0, 0, 1.9292, 1.5442, 1.5442, 1.2641, 1.0661, 1.0661, .9471, .9471, .8, .8; 0, 0, 0, 1.9291, 1.5451, 1.5451, 1.2647, 1.0667, 1.0667, .9484, .9484, .8003, .8003; 0, 0, 0, 1.3197, 1.0944, 1.0944, .93, .8084, .8084, .7386, .7386, .6549, .6549; 0, 0, 0, -.5504, -.5764, -.5764, -.5794, -.5974, -.5974, -.6384, -.6384, -.6414, -.6414; 0, 0, 0, -.7967, -.8179, -.8179, -.815, -.8265, -.8265, -.8695, -.8695, -.8727, -.8727; 0, 0, 0, -.6625, -.6755, -.6755, -.6718, -.678, -.678, -.71, -.71, -.7129, -.7129; 0, 0, 0, -.4372, -.4449, -.4449, -.5659, -.7443, -.7443, -.797, -.797, -.7602, -.7602; 0, 0, 0, -.0005, -.0005, -.0005, -.0005, -.0007, -.0007, -.0008, -.0008, -.0007, -.0007]  Cd_TLU=[.5, .5, .35, .0113, .0094, .0094, .0087, .0065, .0065, .0057, .0057, .0052, .0052; .5, .5, .35, .1226, .1192, .1192, .111, .1087, .1087, .1087, .1087, .1096, .1096; .5, .5, .35, .2813, .2754, .2754, .265, .2622, .2622, .2588, .2588, .2588, .2588; .5, .5, .35, .6981, .6956, .6956, .6919, .6916, .6916, .6764, .6764, .6716, .6716; .5, .5, .35, .6005, .6252, .6252, .6685, .6821, .6821, .654, .654, .6398, .6398; .5, .5, .35, .351, .3709, .3709, .4054, .4161, .4161, .3965, .3965, .3833, .3833; .5, .5, .35, .3293, .3486, .3486, .3824, .3927, .3927, .3737, .3737, .3588, .3588; .5, .5, .35, .3079, .3266, .3266, .3597, .3693, .3693, .3508, .3508, .3341, .3341; .5, .5, .35, .2866, .3047, .3047, .3375, .346, .346, .3275, .3275, .3091, .3091; .5, .5, .35, .2658, .2834, .2834, .3163, .3228, .3228, .3033, .3033, .2835, .2835; .5, .5, .35, .2456, .2625, .2625, .2962, .2991, .2991, .2782, .2782, .2577, .2577; .5, .5, .35, .129, .1313, .1313, .1766, .1275, .1275, .096, .096, .0806, .0806; .5, .5, .35, .119, .1157, .1157, .1621, .1039, .1039, .0709, .0709, .0555, .0555; .5, .5, .35, .1107, .1011, .1011, .143, .0807, .0807, .0494, .0494, .0303, .0303; .5, .5, .35, .1041, .0877, .0877, .123, .0586, .0586, .034, .034, .0152, .0152; .5, .5, .35, .0307, .0145, .0145, .0089, .0068, .0068, .0058, .0058, .0065, .0065; .5, .5, .35, .0156, .0115, .0115, .0106, .013, .013, .013, .013, .0112, .0112; .5, .5, .35, .0194, .0119, .0119, .0123, .0151, .0151, .0146, .0146, .0123, .0123; .5, .5, .35, .0268, .0132, .0132, .0153, .0178, .0178, .0177, .0177, .0135, .0135; .5, .5, .35, .0381, .0154, .0154, .0188, .0252, .0252, .0248, .0248, .0148, .0148; .5, .5, .35, .0563, .019, .019, .0248, .0406, .0406, .0339, .0339, .0365, .0365; .5, .5, .35, .0794, .0262, .0262, .0359, .0587, .0587, .0457, .0457, .0595, .0595; .5, .5, .35, .1104, .0384, .0384, .0602, .077, .077, .0619, .0619, .0823, .0823; .5, .5, .35, .1435, .0591, .0591, .0907, .0982, .0982, .0792, .0792, .1047, .1047; .5, .5, .35, .1813, .0944, .0944, .1213, .1201, .1201, .0973, .0973, .1269, .1269; .5, .5, .35, .2217, .1343, .1343, .1565, .1416, .1416, .1154, .1154, .1491, .1491; .5, .5, .35, .2649, .1779, .1779, .1878, .1632, .1632, .1352, .1352, .1711, .1711; .5, .5, .35, .4382, .3418, .3418, .2921, .2513, .2513, .2194, .2194, .2573, .2573; .5, .5, .35, 1.0687, .884, .884, .7413, .6526, .6526, .6107, .6107, .5307, .5307; .5, .5, .35, 1.1128, .9207, .9207, .7724, .6799, .6799, .6362, .6362, .5527, .5527; .5, .5, .35, 1.8354, 1.5718, 1.5718, 1.3636, 1.232, 1.232, 1.1782, 1.1782, 1.0678, 1.0678; .5, .5, .35, 1.1876, 1.1903, 1.1903, 1.1775, 1.1722, 1.1722, 1.207, 1.207, 1.2112, 1.2112; .5, .5, .35, .7009, .6946, .6946, .6841, .6742, .6742, .6875, .6875, .6898, .6898; .5, .5, .35, .3164, .3083, .3083, .3017, .2929, .2929, .2939, .2939, .2948, .2948; .5, .5, .35, .1294, .1254, .1254, .1229, .1168, .1168, .1143, .1143, .1146, .1146; .5, .5, .35, .0601, .0405, .0405, .0265, .0201, .0201, .0184, .0184, .0197, .0197]  interp_method=simscape.enum.interpolation.linear  extrap_method=simscape.enum.extrapolation.linear  density_spec=foundation.enum.constant_variable.constant  rho=1.225 kg/m^3  rotational_ports=sdl.enum.ConnectionType.Conserving  translational_ports=sdl.enum.ConnectionType.Conserving  model_inertia=true  propeller_inertia=J kg*m^2  propeller_mass=m g  efficiency_sensor=false  n_thr=0.001 Hz  k_thr=0.001  P_thr=0.01 W  operation_check=simscape.enum.assert.action.warn  expose_port_C=0  w_specify=off  w_priority=None  w=0 rad/s  w_nominal_specify=off  w_nominal_unit=rad/s  w_nominal_value=1  Q_specify=off  Q_priority=None  Q=0 N*m  Q_nominal_specify=off  Q_nominal_unit=N*m  Q_nominal_value=1  v_specify=off  v_priority=None  v=0 m/s  v_nominal_specify=off  v_nominal_unit=m/s  v_nominal_value=1  thrust_specify=off  thrust_priority=None  thrust=0 N  thrust_nominal_specify=off  thrust_nominal_unit=N  thrust_nominal_value=1
      settings: InternalSimscapePortConfiguration="{\"Bottom\":[],\"Left\":[{\"id\":\"R1\",\"label\":\"R1\",\"type\":\"foundation.mechanical.rotational.rotational\"}],\"Right\":[{\"id\":\"R2\",\"label\":\"R2\",\"type\":\"foundation.mechanical.translational.translational\"},{\"id\":\"C2\",\"label\":\"C2\",\"type\":\"foundation.mechanical.translational.translational\"}],\"Top\":[]}"
  Electrical Reference1 : fl_lib/Electrical/Electrical Elements/Electrical Reference
  Mechanical Rotational Reference : fl_lib/Mechanical/Rotational Elements/Mechanical Rotational Reference
  Mechanical Translational Reference : fl_lib/Mechanical/Translational Elements/Mechanical Translational Reference
  Motor & Drive (System Level) : ee_lib/Electromechanical/Motor & Drive (System Level)  torque_speed_param=ee.enum.electromech.envelope.torque_power  overtorque_param=ee.enum.electromech.overtorque.no  T_t=[.09, .08, .07, 0] N*m  T_t_intermittent=[.36, .32, .28, 0] N*m  T_t_2D=[.09, .09, .09; .08, .08, .08; .07, .07, .07; 0, 0, 0] N*m  T_t_intermittent_2D=[.36, .36, .36; .32, .32, .32; .28, .28, .28; 0, 0, 0] N*m  w_t=[0, 3750, 7500, 8000] rpm  vdc_t=[6, 12, 24] V  torque_max=1 mN*m  power_max=3 W  torque_max_intermittent=0.4 N*m  power_max_intermittent=120 W  time_overtorque=30 s  time_recover=60 s  Tc=0.02 s  EnableSwitch=simscape.enum.onoff.off  losses_param=1  eff=74  w_eff=3e4 rpm  T_eff=1 mN*m  Piron=0 W  Pbase=0 W  w_eff_vec=[-8000, -4000, 0, 4000, 8000] rpm  T_eff_vec=[0, .03, .06, .09] N*m  v_eff_vec=[100, 250, 400] V  losses_mat=[1.49, 1.67, 2.21, 3.1; .42, .69, 1.14, 2.03; .06, .24, .78, 1.68; .42, .69, 1.14, 2.03; 1.49, 1.67, 2.21, 3.1] W  efficiency_mat=[95, 95, 95, 95; 95, 95, 95, 95; 95, 95, 95, 95; 95, 95, 95, 95; 95, 95, 95, 95]  losses_mat_3D=ones(5, 4, 3) W  efficiency_mat_3D=95 * ones(5, 4, 3)  Res=0 Ohm  enable_fault=simscape.enum.onoff.off  fault_condition=1  fault_threshold=0.5  J=8e-9 kg*m^2  lam=2.5e-8 N*m*s/rad  speed0=0 rpm  faulted_specify=off  faulted_priority=None  faulted=0  faulted_nominal_specify=off  faulted_nominal_unit=1  faulted_nominal_value=1  isSwitchedOff_specify=off  isSwitchedOff_priority=None  isSwitchedOff=0  isSwitchedOff_nominal_specify=off  isSwitchedOff_nominal_unit=1  isSwitchedOff_nominal_value=1  torqueLimitContinuous_specify=off  torqueLimitContinuous_priority=None  torqueLimitContinuous=0 N*m  torqueLimitContinuous_nominal_specify=off  torqueLimitContinuous_nominal_unit=N*m  torqueLimitContinuous_nominal_value=1  alpha=3.93e-3 1/K  Tmeas=25 degC  Tmeas2=125 degC  losses_mat_T2=[1.49, 1.74, 2.49, 3.74; .42, .67, 1.42, 2.67; .06, .31, 1.06, 2.31; .42, .67, 1.42, 2.67; 1.49, 1.74, 2.49, 3.74] W  efficiency_mat_T2=[95, 95, 95, 95; 95, 95, 95, 95; 95, 95, 95, 95; 95, 95, 95, 95; 95, 95, 95, 95]  losses_mat_3D_T2=ones(5, 4, 3) W  efficiency_mat_3D_T2=95 * ones(5, 4, 3)  thermal_mass=100 J/K  initial_temperature=25 degC
  PS-Simulink Converter1 : nesl_utility/PS-Simulink Converter  PhysicalDomain=network_engine_domain  SubClassName=ps_output  LeftPortType=input  RightPortType=output  PseudoPeriodic=off  Frequencies=[]  VectorFormat=inherit  Unit=rpm  AffineConversion=off
  RPM : Display
  Simulink-PS Converter : nesl_utility/Simulink-PS Converter  PhysicalDomain=network_engine_domain  SubClassName=ps_input  LeftPortType=input  RightPortType=output  PseudoPeriodic=off  Frequencies=[]  NoiseDistribution=none  NoiseParameters=[]  Unit=mN*m  AffineConversion=off  FilteringAndDerivatives=provide  SimscapeFilterOrder=1  InputFilterTimeConstant=0.001  UdotUserProvided=0
  R : PMIOPort  Side=Right
  + : PMIOPort  Port=2  Side=Left
  wires:
  PS-Simulink Converter1/1 -> RPM/1  "RPM"
  TC/1 -> Simulink-PS Converter/1
  connections:
  Motor & Drive (System Level)/LConn1 -- +/RConn1
  Simulink-PS Converter/RConn1 -- Motor & Drive (System Level)/LConn2
  R/RConn1 -- Aerodynamic Propeller/RConn1
  Mechanical Translational Reference/LConn1 -- Aerodynamic Propeller/RConn2
  Motor & Drive (System Level)/RConn2 -- PS-Simulink Converter1/LConn1
  Aerodynamic Propeller/LConn1 -- Motor & Drive (System Level)/LConn3
  Electrical Reference1/LConn1 -- Motor & Drive (System Level)/RConn1
  Mechanical Rotational Reference/LConn1 -- Motor & Drive (System Level)/RConn3
